simulink library "AV_Blocks_Library"  (R2018a)
settings: Solver=VariableStepAuto  StartTime=0.0  StopTime=10.0  RelTol=1e-3
undefined symbols (not defined in the file or in its folder): driving
libraries: vdynlib x5, drivinglib x4
settings Model: Creator=chrst  LastModifiedBy=chrst

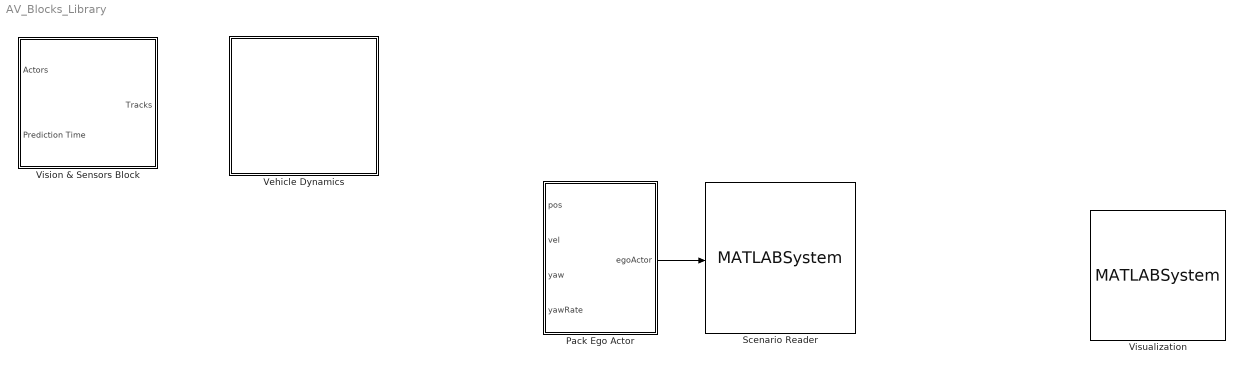
== system AV_Blocks_Library ==
  Pack Ego Actor : MATLAB Function  TreatAsAtomicUnit=on
  Scenario Reader : MATLABSystem  System=AVVerScenarioReader  ScenarioFileName=scenario  EgoActorSource=Input port  EgoActorID=1  RoadBoundaries=on  LaneBoundaries=off  AllBoundaries=off  LaneBoundaryDistance=0:0.5:9.5  LaneBoundaryLocation=center  CurrentLane=off  NumLanes=off  LaneMarkings=off  BusNameSource=Auto  BusName2Source=Auto  BusName3Source=Auto  SimulateUsing=Code generation
      mask Type: AVVerScenarioReader
      mask Display:
      | disp(['Scenario' char(10) 'Reader']);
      | port_label('input',1,'Ego Actor');
      | port_label('output',1,'Actors');
      | port_label('output',2,'Roads');
  Vehicle Dynamics : Subsystem
  Vision & Sensors Block : Subsystem
  Visualization : MATLABSystem  System=AVVerVisualization  XLim=[ 0, 60 ]  YLim=[ -30, 30 ]  HasActors=on  HasVision=off  HasRadar=off  HasTracks=off  TrackPositionSelector=[ 1, 0, 0, 0, 0, 0; 0, 0, 1, 0, 0, 0 ]  TrackVelocitySelector=[ 0, 1, 0, 0, 0, 0; 0, 0, 0, 1, 0, 0 ]  HasMIO=off  HasRoads=off  HasLaneBoundaries=off  HasLaneMarkings=off
      mask Type: AVVerVisualization
      mask Display:
      | disp(['Bird''s-Eye' char(10) 'Plot']);
      | port_label('input',1,'Actors');
  wires:
  Pack Ego Actor/1(egoActor) -> Scenario Reader/1

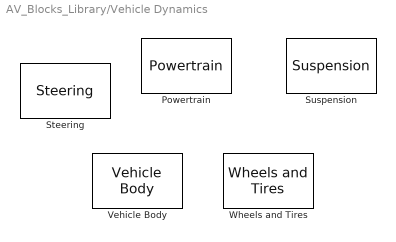
== system AV_Blocks_Library/Vehicle Dynamics ==
  Powertrain : vdynlib/Powertrain  SystemSampleTime=-1
      settings: SourceProductName=Vehicle Dynamics Blockset  SourceProductBaseCode=VE
  Steering : vdynlib/Steering  SystemSampleTime=-1
      settings: SourceProductName=Vehicle Dynamics Blockset  SourceProductBaseCode=VE
  Suspension : vdynlib/Suspension  SystemSampleTime=-1
      settings: SourceProductName=Vehicle Dynamics Blockset  SourceProductBaseCode=VE
  Vehicle Body : vdynlib/Vehicle Body  SystemSampleTime=-1
      settings: SourceProductName=Vehicle Dynamics Blockset  SourceProductBaseCode=VE
  Wheels and Tires : vdynlib/Wheels and Tires  SystemSampleTime=-1
      settings: SourceProductName=Vehicle Dynamics Blockset  SourceProductBaseCode=VE

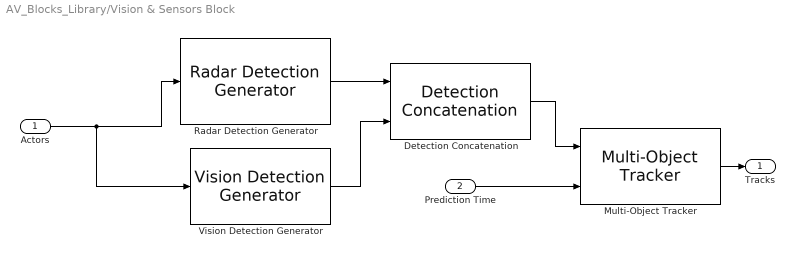
== system AV_Blocks_Library/Vision & Sensors Block ==
  Actors : Inport
  Prediction Time : Inport  Port=2
  Detection Concatenation : drivinglib/Detection Concatenation  NumInputs=2  BusNameSource=Auto  SimulateUsing=Interpreted execution
      settings: SourceProductName=Automated Driving System Toolbox  SourceProductBaseCode=DR
  Multi-Object Tracker : drivinglib/Multi-Object Tracker  FilterInitializationFcn=initcvkf  AssignmentThreshold=30.0  ConfirmationParameters=[ 2, 3 ]  NumCoastingUpdates=5  MaxNumTracks=200  MaxNumSensors=20  TimeInputSource=Input port  HasCostMatrixInput=off  BusNameSource=Auto  TentativeTracksOutputPort=off  AllTracksOutputPort=off  SimulateUsing=Interpreted execution
      settings: SourceProductName=Automated Driving System Toolbox  SourceProductBaseCode=DR
  Radar Detection Generator : drivinglib/Radar Detection Generator  SensorIndex=1  UpdateInterval=0.1  SensorLocation=[ 3.4, 0 ]  Height=0.2  Yaw=0  Pitch=0  Roll=0  BusNameSource=Auto  MaxNumDetectionsSource=Property  MaxNumDetections=50  DetectionCoordinates=Ego Cartesian  SimulateUsing=Interpreted execution  AzimuthResolution=4  ElevationResolution=10  RangeResolution=2.5  RangeRateResolution=0.5  AzimuthBiasFraction=0.1  ElevationBiasFraction=0.1  RangeBiasFraction=0.05  RangeRateBiasFraction=0.05  FieldOfView=[ 20, 5 ]  MaxRange=150  RangeRateLimits=[ -100, 100 ]  DetectionProbability=0.9  FalseAlarmRate=1e-6  ReferenceRange=100  ReferenceRCS=0  HasElevation=off  HasRangeRate=on  HasNoise=on  HasFalseAlarms=on  InitialSeedSource=Repeatable  InitialSeed=0  UsedSeed=driving.internal.SimulinkUtilities.seedManager(gcb)  ActorProfilesSource=Parameters  ActorProfilesParameters=driving.internal.ActorProfilesRadarParameters  ActorProfilesExpression=struct( 'ClassID', 0, 'Length', 4.7, 'Width', 1.8, 'Height', 1.4, 'OriginOffset', [ -1.35, 0, 0 ], 'RCSPattern', [ 10, 10; 10, 10 ], 'RCSAzimuthAngles', [ -180, 180 ], 'RCSElevationAngles', [ -90, 90 ] )
      settings: SourceProductName=Automated Driving System Toolbox  SourceProductBaseCode=DR
  Vision Detection Generator : drivinglib/Vision Detection Generator  SensorIndex=1  DetectorOutput=Objects only  UpdateInterval=0.1  LaneUpdateInterval=0.1  SensorLocation=[ 1.9, 0 ]  Height=1.1  Yaw=0  Pitch=1  Roll=0  BusNameSource=Auto  BusName2Source=Auto  MaxNumDetectionsSource=Property  MaxNumDetections=50  MaxNumLanesSource=Property  MaxNumLanes=30  DetectionCoordinates=Ego Cartesian  SimulateUsing=Interpreted execution  MaxRange=150  BoundingBoxAccuracy=5  ProcessNoiseIntensity=5  MaxSpeed=50  MaxAllowedOcclusion=0.5  MinObjectImageSize=[ 15, 15 ]  DetectionProbability=0.9  FalsePositivesPerImage=0.1  MinLaneImageSize=[ 20, 3 ]  LaneBoundaryAccuracy=3  HasNoise=on  InitialSeedSource=Repeatable  InitialSeed=0  UsedSeed=driving.internal.SimulinkUtilities.seedManager(gcb)  ActorProfilesSource=Parameters  ActorProfilesParameters=driving.internal.ActorProfilesParameters  ActorProfilesExpression=struct( 'ClassID', 0, 'Length', 4.7, 'Width', 1.8, 'Height', 1.4, 'OriginOffset', [ -1.35, 0, 0 ] )  Intrinsics=driving.internal.cameraIntrinsics
      settings: SourceProductName=Automated Driving System Toolbox  SourceProductBaseCode=DR
  Tracks : Outport
  wires:
  Actors/1 -> Vision Detection Generator/1, Radar Detection Generator/1
  Prediction Time/1 -> Multi-Object Tracker/2
  Radar Detection Generator/1 -> Detection Concatenation/1
  Vision Detection Generator/1 -> Detection Concatenation/2
  Detection Concatenation/1 -> Multi-Object Tracker/1
  Multi-Object Tracker/1 -> Tracks/1

== matlab function AV_Blocks_Library/Pack Ego Actor ==
  data: pos input; egoActor output; vel input; yaw input; yawRate input
function egoActor = packEgo(pos,vel,yaw,yawRate)
% Pack ego information into a single ego actor bus
%
% Imoprtant note:
% Output is a bus of type BusActorsActors. This is the same bus used by the
% helperScenarioReader to output an individual actor. If you change the
% output bus name of helperScenarioReader, change the output bus name here
% as well by clicking on 'Edit Data' in the menu above.

egoActor = struct(...
    'ActorID',1,...
    'Position', [pos(1) pos(2) 0], ...
    'Velocity', [vel(1) vel(2) 0], ...
    'Roll', 0, ...
    'Pitch', 0, ...
    'Yaw', yaw, ...
    'AngularVelocity', [0 0 yawRate]);
